simulink model "gm_echo_8b"  (R2018a)
settings: Solver=VariableStepAuto  StartTime=0.0  StopTime=7.5  RelTol=1e-3
libraries: dspvision x2
settings Model: Creator=Lu  LastModifiedBy=Lu
settings OptimizationCC: BlockReduction=off  ConditionallyExecuteInputs=off
settings DebuggingCC: InheritedTsInSrcMsg=none

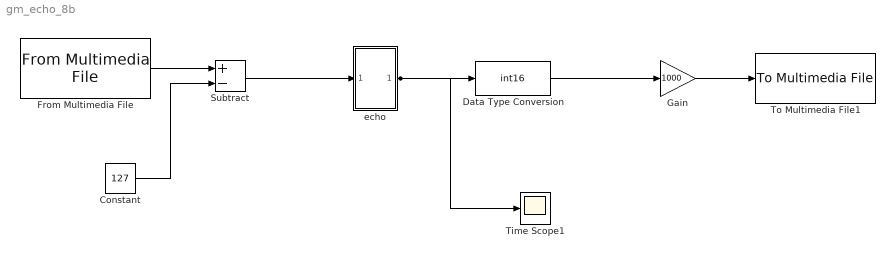
== system gm_echo_8b ==
  Constant : Constant  Value=127  OutDataTypeStr=int8
  Data Type Conversion : DataTypeConversion  OutDataTypeStr=int16
  From Multimedia File : dspvision/From Multimedia File  inputFilename=C:\Users\lugfe\Documents\GitHub\dsp-fpgay\TP FINAL\audio effects\dialog05_8b.wav  loop=on  numPlays=1  outputStreams=Audio only  videoDataType=single  audioDataType=uint8  inheritSampleTime=on  userDefinedSampleTime=1/30  noAudioOutput=off  isIntensityVideo=off  fourcc=RGB  colorVideoFormat=Separate color signals  outputEOF=off  dataOrg=Column-major  audioFrameSize=1  computeAudioFrameSize=off  outSamplingMode=Sample based
      settings: SourceProductBaseCode=VP
  Gain : Gain  Gain=1000  OutDataTypeStr=int16  SaturateOnIntegerOverflow=on
  Subtract : Sum  Inputs=+-  AccumDataTypeStr=int8  OutDataTypeStr=int8
  Time Scope1 : Scope
  To Multimedia File1 : dspvision/To Multimedia File  outputFilename=C:\Users\lugfe\Documents\GitHub\dsp-fpgay\TP FINAL\audio effects\delay_little-wing.wav  streamSelection=Audio only  videoCompressor=None (uncompressed)  audioCompressor=None (uncompressed)  imagePorts=Separate color signals  fileType=WAV  audioDatatype=Determine from input data type  fourcc=RGB  videoQuality=75  mj2000CompFactor=10
      settings: SourceProductName=Computer Vision System Toolbox  SourceProductBaseCode=VP
  echo : Subsystem
  wires:
  Gain/1 -> To Multimedia File1/1
  From Multimedia File/1 -> Subtract/1
  Constant/1 -> Subtract/2
  Subtract/1 -> echo/1(In1)
  echo/1(Out1) -> Time Scope1/1, Data Type Conversion/1
  Data Type Conversion/1 -> Gain/1

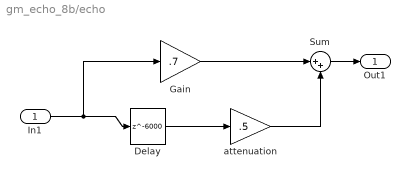
== system gm_echo_8b/echo ==
  In1 : Inport  OutDataTypeStr=int8
  Delay : Delay  DelayLength=6000  DelayLengthUpperLimit=10000  InitialCondition=0  InputProcessing=Columns as channels (frame based)
  Gain : Gain  Gain=.7  ParamDataTypeStr=int16  OutDataTypeStr=int8
  Sum : Sum  Inputs=|++
  attenuation : Gain  Gain=.5  OutDataTypeStr=int8  RndMeth=Round
  Out1 : Outport
  wires:
  Delay/1 -> attenuation/1
  Sum/1 -> Out1/1
  Gain/1 -> Sum/1
  attenuation/1 -> Sum/2
  In1/1 -> Gain/1, Delay/1
